simulink model "psbswitch"  (Simulink 6.0)
settings: Solver=ode15s  SolverMode=SingleTasking  StartTime=0.0  StopTime=0.2  RelTol=1e-3  AbsTol=1e-3
libraries: powerlib2 x11, powerlib_extras x1
settings Model: Creator=patrice  LastModifiedBy=batserve  ExtModeTrigMode=oneshot  ExtModeArmWhenConnect=off  ExtModeAutoUpdateStatusClock=off
settings SolverCC: MaxOrder=4
settings DataIOCC: LimitDataPoints=off  SignalLoggingName=sigsOut
settings OptimizationCC: BlockReduction=off  BooleanDataType=off
settings DebuggingCC: SolverPrmCheckMsg=none
settings HardwareCC: TargetUnknown=on
settings RTWCC: TemplateMakefile=grt_unix.tmf

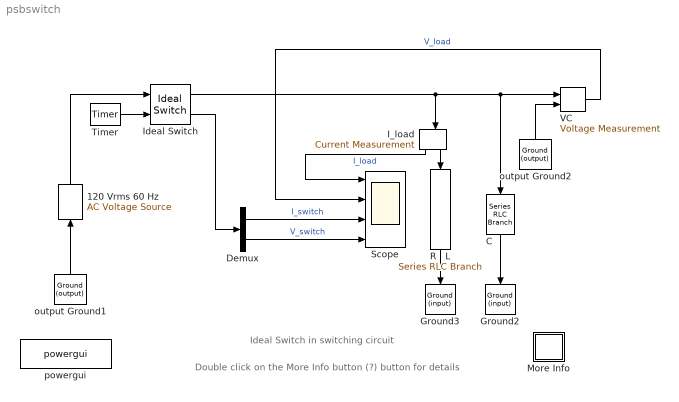
== system psbswitch ==
  note: Double click on the More Info button (?) button for details
  note: Ideal Switch in switching circuit
  120 Vrms 60 Hz : powerlib2/Electrical Sources/AC Voltage Source  Tag=PoWeRsYsTeMbLoCk  Orientation=up  A=120*sqrt(2)  P=0  F=60  stime=0  mesure=None  PSBOutputType=1
  C : powerlib2/Elements/Series RLC Branch  Tag=PoWeRsYsTeMbLoCk  Orientation=down  a=0  b=0  c=10e-6  mesure=None  PSBOutputType=1
  Demux : Demux  Outputs=2
  Ground2 : powerlib2/Connectors/Ground (input)  Tag=PoWeRsYsTeMbLoCk  Orientation=down
  Ground3 : powerlib2/Connectors/Ground (input)  Tag=PoWeRsYsTeMbLoCk  Orientation=down
  I_load : powerlib2/Measurements/Current Measurement  Tag=PoWeRsYsTeMmEaSuReMeNt  Orientation=down  PhasorSimulation=off  OutputType=Magnitude  PSBOutputType=01  PSBequivalent=0
  Ideal Switch : powerlib2/Power Electronics/Ideal Switch  Tag=PoWeRsYsTeMbLoCk  Ron=0.01  Lon=1e-9  IC=1  Rs=inf  Cs=0.1e-6  PSBOutputType=10
  More Info : Subsystem
      mask Display: disp('?')
  R   L : powerlib2/Elements/Series RLC Branch  Tag=PoWeRsYsTeMbLoCk  Orientation=down  a=10  b=.1  c=inf  mesure=None  PSBOutputType=1
  Scope : Scope  NumInputPorts=4
      settings: TimeRange=0.2  YMin=-20~-1500~-10.20144628099172~-2000  YMax=15~1500~10.18706564613074~2000  DataFormat=Array
  Timer : powerlib_extras/Control  Blocks/Timer  t="[0 3/60  8.25/60 ]"  e=[1 0 1]
  VC : powerlib2/Measurements/Voltage Measurement  Tag=PoWeRsYsTeMmEaSuReMeNt  PhasorSimulation=off  OutputType=Magnitude  PSBOutputType=0  PSBequivalent=0
  output Ground1 : powerlib2/Connectors/Ground (output)  Tag=PoWeRsYsTeMbLoCk  Orientation=up  PSBOutputType=1
  output Ground2 : powerlib2/Connectors/Ground (output)  Tag=PoWeRsYsTeMbLoCk  Orientation=up  PSBOutputType=1
  powergui : powerlib2/powergui  Frange=logspace(0,3,50)  Ylog=off  Xlog=off  save=off  variable=ZData  ZoomFFT=on  StartTime=0.0  cycles=1  DisplayStyle=off  fundamental=60  FreqAxis=off  MaxFrequency=1000  frequencyindice=1  frequencyindicesteady=1  RmsSteady=1  display=off  Ts=0  methode=off  frequency=60  echomessages=off
  wires:
  Timer/1 -> Ideal Switch/2
  120 Vrms 60 Hz/1 -> Ideal Switch/1
  output Ground1/1 -> 120 Vrms 60 Hz/1
  Ideal Switch/2 -> Demux/1
  R   L/1 -> Ground3/1
  C/1 -> Ground2/1
  output Ground2/1 -> VC/2
  I_load/2 -> R   L/1
  Ideal Switch/1 -> I_load/1, C/1, VC/1
  I_load/1 -> Scope/1  "I_load"
  VC/1 -> Scope/2  "V_load"
  Demux/1 -> Scope/3  "I_switch"
  Demux/2 -> Scope/4  "V_switch"

== system psbswitch/More Info ==
  note: The Ideal Switch is used to switch  an  RLC load on a 120V rms, 60 Hz voltage source.
      | The switch is initially closed.
      | It is  turned off  at t = 3 cycles (50 ms), then it is reclosed at t = 8.25 cycles (138 ms).
  note: This example illustrates the use of the Ideal Switch
      | ____________________________________________
  note: Observe that current chopping produces a load overvoltage at switch opening.
      | Also observe high switch curent spike when the capacitive circuit is re-energized at maximum source voltage.
